simulink model "Three-phase Asynchronous Motor_FR Rotation"  (R2017b)
settings: Solver=ode23  StartTime=0.0  StopTime=2.5  MaxStep=1e-4  RelTol=1e-3
libraries: powerlib x7
settings Model: Creator=13248  LastModifiedBy=13248

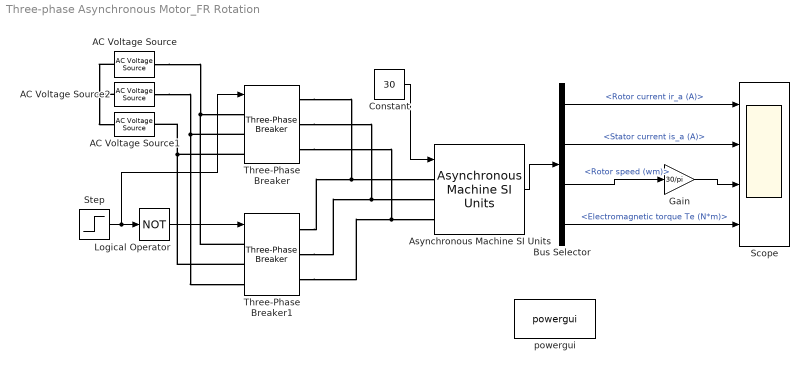
== system Three-phase Asynchronous Motor_FR Rotation ==
  AC Voltage Source : powerlib/Electrical Sources/AC Voltage Source  Amplitude=400  Phase=0  Frequency=50  SampleTime=0  Measurements=None  BusType=swing  Pref=10e3  Qref=0  Qmin=-inf  Qmax=+inf
  AC Voltage Source1 : powerlib/Electrical Sources/AC Voltage Source  Amplitude=400  Phase=-120  Frequency=50  SampleTime=0  Measurements=None  BusType=swing  Pref=10e3  Qref=0  Qmin=-inf  Qmax=+inf
  AC Voltage Source2 : powerlib/Electrical Sources/AC Voltage Source  Amplitude=400  Phase=120  Frequency=50  SampleTime=0  Measurements=None  BusType=swing  Pref=10e3  Qref=0  Qmin=-inf  Qmax=+inf
  Asynchronous Machine SI Units : powerlib/Machines/Asynchronous Machine SI Units  RotorType=Squirrel-cage  PresetModel="20:  150 HP (110KW) 400 V 50Hz 1487 RPM"  MechanicalLoad=Torque Tm  ShowDetailedParameters=on  ReferenceFrame=Rotor  Units=SI  MeasurementBus=off  NominalParameters=[1.1e+05 400 50]  Stator=[0.02155 0.000226]  Rotor=[0.01231 0.000226]  Cage1=[0.4155 0.002066]  Cage2=[0.4168 0.0003495]  Lm=0.01038  Mechanical=[2.3 0.05421 2]  PolePairs=2  InitialConditions=[0 0 0 0 0 0 0 0]  SimulateSaturation=off  Saturation=[14.03593122, 27.81365428, 53.79336849, 72.68890987, 97.98006896, 148.6815601, 215.7428561, 302.9841135, 428.7778367 ; 230, 322, 414, 460, 506, 552, 598, 644, 690]  LoadFlowParameters=1492000  TsPowergui=0  TsBlock=-1  IterativeModel=Trapezoidal non iterative  IterativeDiscreteModel=Trapezoidal non iterative  Pmec=1.492e+006
  Bus Selector : BusSelector  OutputSignals=Rotor measurements.Rotor current ir_a (A),Stator measurements.Stator current is_a (A),Mechanical.Rotor speed (wm),Mechanical.Electromagnetic torque Te (N*m)
  Constant : Constant  Value=30
  Gain : Gain  Gain=30/pi
  Logical Operator : Logic  Operator=NOT  AllPortsSameDT=off  OutDataTypeStr=boolean
  Scope : Scope  NumInputPorts=4
  Step : Step  SampleTime=0
  Three-Phase Breaker : powerlib/Elements/Three-Phase Breaker  InitialState=open  SwitchA=on  SwitchB=on  SwitchC=on  SwitchTimes="[1/60  5/60]"  External=on  BreakerResistance=0.01  SnubberResistance=1e6  SnubberCapacitance=inf  Measurements=None
  Three-Phase Breaker1 : powerlib/Elements/Three-Phase Breaker  InitialState=open  SwitchA=on  SwitchB=on  SwitchC=on  SwitchTimes="[1/60  5/60]"  External=on  BreakerResistance=0.01  SnubberResistance=1e6  SnubberCapacitance=inf  Measurements=None
  powergui : powerlib/powergui  Priority=1  SimulationMode=Continuous  SampleTime=50e-6  frequency=60  Iterations=50  frequencyindice=50  Pbase=100e6  ErrMax=1e-4  UnitsV=kV  UnitsW=MW  buscounter=0  FunctionMessages=off  echomessages=off  EnableUseOfTLC=off  CurrentSourceSwitches=off  DisableSnubberDevices=off  DisableRonSwitches=off  DisableVfSwitches=off  DisplayEquations=off  SolverType=Tustin/Backward Euler (TBE)  Interpol=off  ExternalGateDelay=off  methode=off  Ts=100  x0status=blocks  SPID=on  SwTol=0  HookPort=off  RestoreLinks=warning  ResistiveCurrentMeasurement=off  Frange=[0:2:500]  Ylog=off  Xlog=on  ShowGrid=off  save=off  variable=ZData  structure=0  ZoomFFT=off  StartTime=0.0  cycles=1  DisplayStyle=1  fundamental=60  FreqAxis=off  MaxFrequency=1000  frequencyindicesteady=1  RmsSteady=1  display=off
  wires:
  Asynchronous Machine SI Units/1 -> Bus Selector/1
  Bus Selector/3 -> Gain/1  "<Rotor speed (wm)>"
  Bus Selector/4 -> Scope/4  "<Electromagnetic torque Te (N*m)>"
  Bus Selector/1 -> Scope/1  "<Rotor current ir_a (A)>"
  Bus Selector/2 -> Scope/2  "<Stator current is_a (A)>"
  Constant/1 -> Asynchronous Machine SI Units/1
  Step/1 -> Logical Operator/1, Three-Phase Breaker/1
  Logical Operator/1 -> Three-Phase Breaker1/1
  Gain/1 -> Scope/3
  connections:
  Three-Phase Breaker1/RConn3 -- Three-Phase Breaker/RConn3 -- Asynchronous Machine SI Units/LConn3
  Three-Phase Breaker1/RConn2 -- Three-Phase Breaker/RConn2 -- Asynchronous Machine SI Units/LConn2
  Three-Phase Breaker1/RConn1 -- Three-Phase Breaker/RConn1 -- Asynchronous Machine SI Units/LConn1
  AC Voltage Source/LConn1 -- AC Voltage Source2/LConn1 -- AC Voltage Source1/LConn1
  AC Voltage Source/RConn1 -- Three-Phase Breaker/LConn1 -- Three-Phase Breaker1/LConn1
  AC Voltage Source2/RConn1 -- Three-Phase Breaker/LConn2 -- Three-Phase Breaker1/LConn3
  Three-Phase Breaker1/LConn2 -- Three-Phase Breaker/LConn3 -- AC Voltage Source1/RConn1
